simulink model "MinimumJerkPlanner"  (R2024b)
settings: configuration reference "MCConfiguration" (kept outside this file)
undefined symbols (not defined in the file): acc_max, bVelocityMove, InitTrajectory, p0, pos_max, pos_min, target_pos, target_vel, Trajectory_set_pos_end, Trajectory_set_pos_raw, Trajectory_velocity_stop, Ts, vA, vel_max, velAvg, vK0, vK1, vK2, vK3, vK4, vK5, vK6, vT, vTimer, vV, vX, xA, xK0, xK1, xK2, xK3, xK4, xK5, xStar, xT, xTimer, xV, xX
libraries: simulink x4, shareduavrstlib x2
settings Model: DataDictionary=MotionController.sldd  Creator=rpumpo  LastModifiedBy=rpumpo
settings ConfigSetRef: SourceName=MCConfiguration

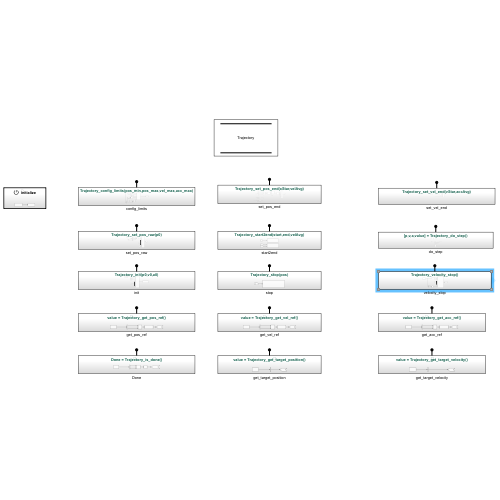
[thumbnail: Simulink's stored preview of the top-level diagram]
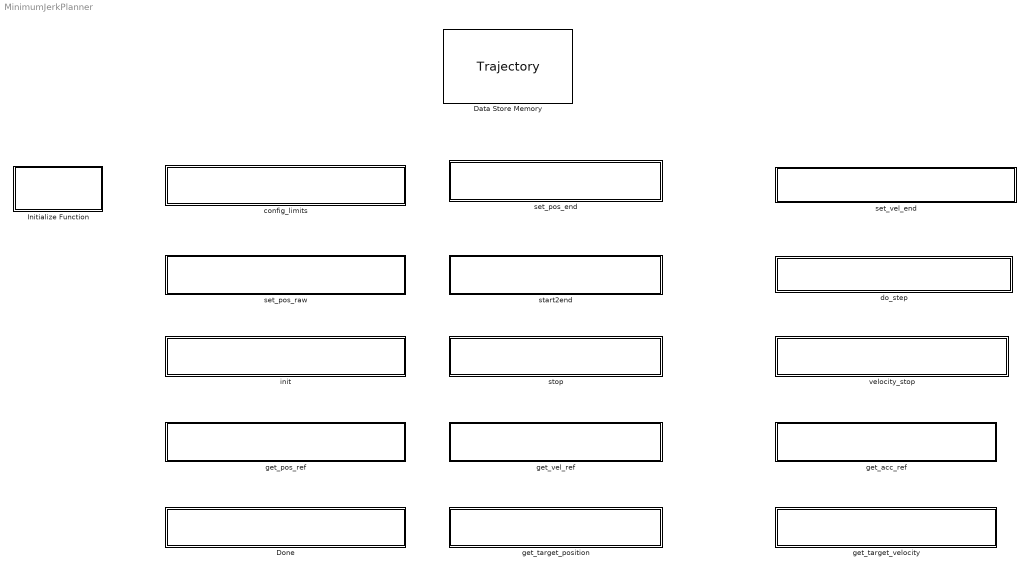
== system MinimumJerkPlanner ==
  Data Store Memory : DataStoreMemory  DataStoreName=Trajectory  WriteAfterWriteMsg=warning  ShowAdditionalParam=off  OutDataTypeStr=Bus: trajectoryhidParameters
  Done : Subsystem  TreatAsAtomicUnit=on
  Initialize Function : Subsystem  TreatAsAtomicUnit=on
  config_limits : Subsystem  TreatAsAtomicUnit=on
  do_step : Subsystem  TreatAsAtomicUnit=on
  get_acc_ref : Subsystem  TreatAsAtomicUnit=on
  get_pos_ref : Subsystem  TreatAsAtomicUnit=on
  get_target_position : Subsystem  TreatAsAtomicUnit=on
  get_target_velocity : Subsystem  TreatAsAtomicUnit=on
  get_vel_ref : Subsystem  TreatAsAtomicUnit=on
  init : Subsystem  TreatAsAtomicUnit=on
  set_pos_end : Subsystem  TreatAsAtomicUnit=on
  set_pos_raw : Subsystem  TreatAsAtomicUnit=on
  set_vel_end : Subsystem  TreatAsAtomicUnit=on
  start2end : Subsystem  TreatAsAtomicUnit=on
  stop : Subsystem  TreatAsAtomicUnit=on
  velocity_stop : Subsystem  TreatAsAtomicUnit=on

== system MinimumJerkPlanner/Done ==
  Trajectory_is_done : TriggerPort  TriggerType=function-call  IsSimulinkFunction=on  FunctionName=Trajectory_is_done  FunctionVisibility=scoped  VariantControl=(inherit)
  Add : Sum  Inputs=+-
  Bus Selector : BusSelector  OutputSignals=xTimer,xT
  Compare To Constant : simulink/Logic and Bit Operations/Compare To Constant  relop=>=  const=0  OutDataTypeStr=boolean
  Data Store Read : DataStoreRead  DataStoreName=Trajectory  IndexOptions=Index vector (dialog)  Indices=1  OutputSizes=1
  Done : ArgOut  OutDataTypeStr=boolean  ArgumentName=Done
  wires:
  Data Store Read/1 -> Bus Selector/1
  Bus Selector/2 -> Add/2  "<xT>"
  Bus Selector/1 -> Add/1  "<xTimer>"
  Add/1 -> Compare To Constant/1
  Compare To Constant/1 -> Done/1

== system MinimumJerkPlanner/Initialize Function ==
  Constant : Constant  Value=InitTrajectory  OutDataTypeStr=Bus: trajectoryhidParameters
  Data Store Write : DataStoreWrite  DataStoreName=Trajectory  IndexOptions=Index vector (dialog)  Indices=1  OutputSizes=1
  Event Listener : EventListener  DisableCoverage=on  EventName=reset
  wires:
  Constant/1 -> Data Store Write/1

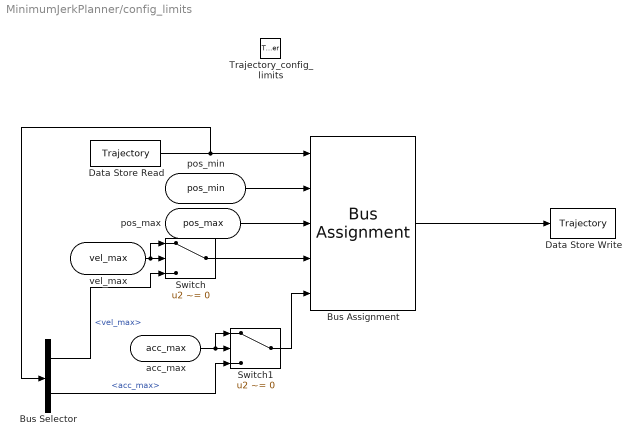
== system MinimumJerkPlanner/config_limits ==
  Trajectory_config_limits : TriggerPort  TriggerType=function-call  IsSimulinkFunction=on  FunctionName=Trajectory_config_limits  FunctionVisibility=scoped  VariantControl=(inherit)
  Bus Assignment : BusAssignment  AssignedSignals=pos_min,pos_max,vel_max,acc_max
  Bus Selector : BusSelector  OutputSignals=vel_max,acc_max
  Data Store Read : DataStoreRead  DataStoreName=Trajectory  IndexOptions=Index vector (dialog)  Indices=1  OutputSizes=1
  Data Store Write : DataStoreWrite  DataStoreName=Trajectory  IndexOptions=Index vector (dialog)  Indices=1  OutputSizes=1
  Switch : Switch  Criteria=u2 ~= 0  SaturateOnIntegerOverflow=off  InputSameDT=off
  Switch1 : Switch  Criteria=u2 ~= 0  SaturateOnIntegerOverflow=off  InputSameDT=off
  pos_min : ArgIn  OutDataTypeStr=single  ArgumentName=pos_min
  pos_max : ArgIn  Port=2  OutDataTypeStr=single  ArgumentName=pos_max
  vel_max : ArgIn  Port=3  OutDataTypeStr=single  ArgumentName=vel_max
  acc_max : ArgIn  Port=4  OutDataTypeStr=single  ArgumentName=acc_max
  wires:
  Data Store Read/1 -> Bus Selector/1, Bus Assignment/1
  pos_min/1 -> Bus Assignment/2
  pos_max/1 -> Bus Assignment/3
  Bus Assignment/1 -> Data Store Write/1
  vel_max/1 -> Switch/1, Switch/2
  Bus Selector/1 -> Switch/3  "<vel_max>"
  Switch/1 -> Bus Assignment/4
  acc_max/1 -> Switch1/1, Switch1/2
  Bus Selector/2 -> Switch1/3  "<acc_max>"
  Switch1/1 -> Bus Assignment/5

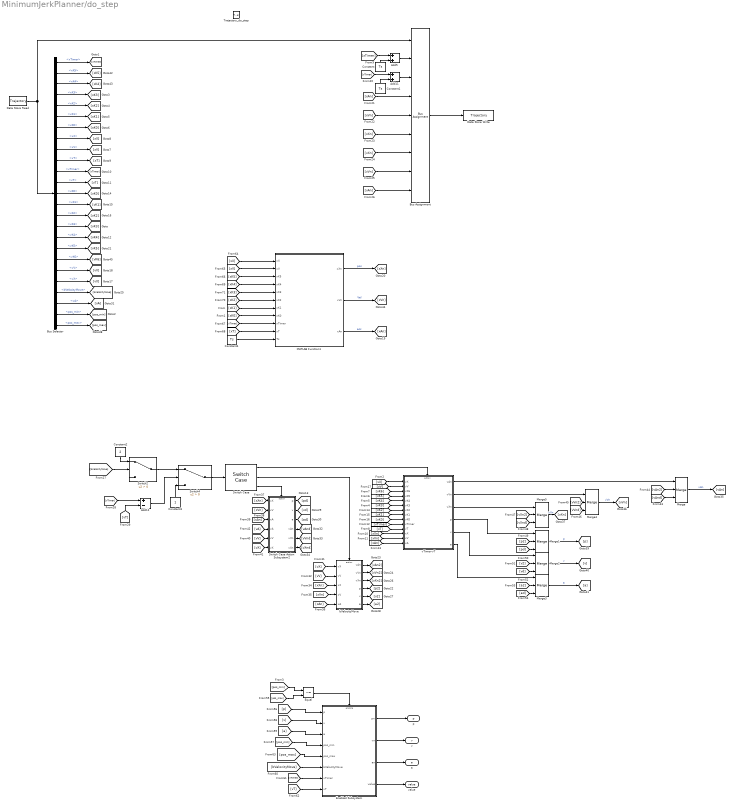
== system MinimumJerkPlanner/do_step ==
  Trajectory_do_step : TriggerPort  TriggerType=function-call  IsSimulinkFunction=on  FunctionName=Trajectory_do_step  FunctionVisibility=scoped  VariantControl=(inherit)
  Add11 : Sum
  Add12 : Sum  Inputs=+-
  Add5 : Sum
  Bus Assignment : BusAssignment  AssignedSignals=xTimer,vTimer,xA,xV,xX,vX,vV,vA
  Bus Selector : BusSelector  OutputSignals=xTimer,xK5,xK4,xK3,xK2,xK1,xK0,xX,xV,xT,vTimer,vT,vK0,vK1,vK2,vK3,vK4,vK5,vK6,vV,vX,bVelocityMove,vA,pos_min,pos_max
  Constant : Constant  Value=Ts  OutDataTypeStr=single
  Constant1 : Constant  Value=Ts  OutDataTypeStr=single
  Constant2 : Constant  Value=2
  Constant3 : Constant
  Constant4 : Constant  Value=Ts  OutDataTypeStr=single
  Data Store Read : DataStoreRead  DataStoreName=Trajectory  IndexOptions=Index vector (dialog)  Indices=1  OutputSizes=1
  Data Store Write : DataStoreWrite  DataStoreName=Trajectory  IndexOptions=Index vector (dialog)  Indices=1  OutputSizes=1
  Enabled Subsystem : Subsystem  TreatAsAtomicUnit=on
  Equal : RelationalOperator  Operator=~=  OutDataTypeStr=boolean  RndMeth=Simplest  InputSameDT=off
  MATLAB Function1 : MATLAB Function  TreatAsAtomicUnit=on
  Merge{,1..5} (6 alike) : Merge  Inputs=3
  Switch Case : SwitchCase  CaseConditions={1,2}
  Switch Case Action Subsystem2 : Subsystem  TreatAsAtomicUnit=on
  Switch2 : Switch  Criteria=u2 > Threshold  SaturateOnIntegerOverflow=off  InputSameDT=off
  Switch4 : Switch  Criteria=u2 > Threshold  SaturateOnIntegerOverflow=off  InputSameDT=off
  bVelocityMove : Subsystem  TreatAsAtomicUnit=on
  vTimer-vT : Subsystem  TreatAsAtomicUnit=on
  p : ArgOut  DisableCoverage=on  OutDataTypeStr=single  ArgumentName=p
  v : ArgOut  DisableCoverage=on  Port=2  OutDataTypeStr=single  ArgumentName=v
  a : ArgOut  DisableCoverage=on  Port=3  OutDataTypeStr=single  ArgumentName=a
  value : ArgOut  DisableCoverage=on  Port=4  OutDataTypeStr=int32  ArgumentName=value
  wires:
  Data Store Read/1 -> Bus Assignment/1, Bus Selector/1
  Bus Selector/1 -> [xTimer]  "<xTimer>"
  Bus Selector/4 -> [xK3]  "<xK3>"
  Bus Selector/5 -> [xK2]  "<xK2>"
  Bus Selector/6 -> [xK1]  "<xK1>"
  Bus Selector/7 -> [xK0]  "<xK0>"
  Bus Selector/8 -> [xX]  "<xX>"
  Bus Selector/9 -> [xV]  "<xV>"
  [xTimer] -> Add5/1
  Constant/1 -> Add5/2
  Add5/1 -> Bus Assignment/2
  Bus Assignment/1 -> Data Store Write/1
  Bus Selector/10 -> [xT]  "<xT>"
  Bus Selector/11 -> [vTimer]  "<vTimer>"
  Bus Selector/12 -> [vT]  "<vT>"
  Bus Selector/13 -> [vK0]  "<vK0>"
  Bus Selector/14 -> [vK1]  "<vK1>"
  Bus Selector/15 -> [vK2]  "<vK2>"
  Bus Selector/20 -> [vV]  "<vV>"
  Bus Selector/21 -> [vX]  "<vX>"
  [xAn] -> Bus Assignment/4
  [xVn] -> Bus Assignment/5
  [xXn] -> Bus Assignment/6
  [vXn] -> Bus Assignment/7
  [vVn] -> Bus Assignment/8
  [vAn] -> Bus Assignment/9
  Bus Selector/22 -> [bVelocityMove]  "<bVelocityMove>"
  [bVelocityMove] -> Switch2/2
  Constant2/1 -> Switch2/1
  Switch Case/1 -> vTimer-vT/Action
  Switch Case/2 -> bVelocityMove/Action
  Switch2/1 -> Switch4/1
  [vX] -> bVelocityMove/1(vX)
  [vV] -> bVelocityMove/2(vV)
  [vTimer] -> Add12/1
  [vT] -> Add12/2
  Add12/1 -> Switch4/2
  Constant3/1 -> Switch4/3
  Switch4/1 -> Switch Case/1
  [vTimer] -> vTimer-vT/10(vTimer)
  [vX] -> vTimer-vT/1(vX)
  [vK2] -> vTimer-vT/7(vK2)
  [vK1] -> vTimer-vT/8(vK1)
  [vK0] -> vTimer-vT/9(vK0)
  [vV] -> vTimer-vT/2(vV)
  [vTimer] -> Add11/1
  Constant1/1 -> Add11/2
  Add11/1 -> Bus Assignment/3
  [xXn] -> bVelocityMove/3(xX)
  [xVn] -> bVelocityMove/4(xV)
  [xAn] -> bVelocityMove/5(xA)
  Switch Case/3 -> Switch Case Action Subsystem2/Action
  [xXn] -> Switch Case Action Subsystem2/1(xX)
  [xVn] -> Switch Case Action Subsystem2/2(xV)
  [xAn] -> Switch Case Action Subsystem2/3(xA)
  Merge/1 -> [vAn]  "vAn"
  Merge1/1 -> [p]  "p"
  [vV] -> Switch Case Action Subsystem2/5(vV)
  [vX] -> Switch Case Action Subsystem2/6(vX)
  [vA] -> Switch Case Action Subsystem2/4(vA)
  Switch Case Action Subsystem2/1(p) -> [pd]
  bVelocityMove/4(p) -> [p2]
  vTimer-vT/4(p) -> Merge1/1
  vTimer-vT/5(v) -> Merge2/1
  vTimer-vT/6(a) -> Merge3/1
  bVelocityMove/6(a) -> [a2]
  bVelocityMove/5(v) -> [v2]
  Switch Case Action Subsystem2/2(v) -> [vd]
  Switch Case Action Subsystem2/3(a) -> [ad]
  Bus Selector/23 -> [vA]  "<vA>"
  vTimer-vT/1(vAn) -> Merge/1
  [vAnd] -> Merge/3
  [vAn2] -> Merge/2
  bVelocityMove/1(vAn) -> [vAn2]
  bVelocityMove/2(vVn) -> [vVn2]
  bVelocityMove/3(vXn) -> [vXn2]
  Switch Case Action Subsystem2/4(vAn) -> [vAnd]
  Switch Case Action Subsystem2/5(vVn) -> [vVnd]
  Switch Case Action Subsystem2/6(vXn) -> [vXnd]
  vTimer-vT/2(vVn) -> Merge4/1
  [vVn2] -> Merge4/2
  [vVnd] -> Merge4/3
  Merge4/1 -> [vVn]  "vVn"
  vTimer-vT/3(vXn) -> Merge5/1
  Merge5/1 -> [vXn]  "vXn"
  [vXn2] -> Merge5/2
  [vXnd] -> Merge5/3
  [p2] -> Merge1/2
  [pd] -> Merge1/3
  [v2] -> Merge2/2
  [vd] -> Merge2/3
  [a2] -> Merge3/2
  [ad] -> Merge3/3
  Bus Selector/24 -> [pos_min]  "<pos_min>"
  Bus Selector/25 -> [pos_max]  "<pos_max>"
  [pos_min] -> Equal/1
  [pos_max] -> Equal/2
  Equal/1 -> Enabled Subsystem/Enable
  [p] -> Enabled Subsystem/1(p)
  [pos_min] -> Enabled Subsystem/4(pos_min)
  Merge2/1 -> [v]  "v"
  Merge3/1 -> [a]  "a"
  [v] -> Enabled Subsystem/2(v)
  [a] -> Enabled Subsystem/3(a)
  [bVelocityMove] -> Enabled Subsystem/6(bVelocityMove)
  [vTimer] -> Enabled Subsystem/7(vTimer)
  [vT] -> Enabled Subsystem/8(vT)
  [pos_max] -> Enabled Subsystem/5(pos_max)
  Enabled Subsystem/2(vn) -> v/1
  Enabled Subsystem/3(an) -> a/1
  Enabled Subsystem/1(pn) -> p/1
  Enabled Subsystem/4(value) -> value/1
  Bus Selector/2 -> [xK5]  "<xK5>"
  Bus Selector/3 -> [xK4]  "<xK4>"
  [xX] -> MATLAB Function1/1(xX)
  [xV] -> MATLAB Function1/2(xV)
  [xK5] -> MATLAB Function1/3(xK5)
  MATLAB Function1/2(xVn) -> [xVn]  "Vel"
  [xTimer] -> MATLAB Function1/9(xTimer)
  [xT] -> MATLAB Function1/10(xT)
  [xK4] -> MATLAB Function1/4(xK4)
  [xK3] -> MATLAB Function1/5(xK3)
  [xK2] -> MATLAB Function1/6(xK2)
  Constant4/1 -> MATLAB Function1/11(Ts)
  [xK1] -> MATLAB Function1/7(xK1)
  [xK0] -> MATLAB Function1/8(xK0)
  MATLAB Function1/3(xAn) -> [xAn]  "acc"
  MATLAB Function1/1(xXn) -> [xXn]  "pos"
  [vK6] -> vTimer-vT/3(vK6)
  [vK5] -> vTimer-vT/4(vK5)
  [vK4] -> vTimer-vT/5(vK4)
  [vK3] -> vTimer-vT/6(vK3)
  [vT] -> vTimer-vT/11(vT)
  [xXn] -> vTimer-vT/12(xX)
  [xVn] -> vTimer-vT/13(xV)
  [xAn] -> vTimer-vT/14(xA)
  Bus Selector/16 -> [vK3]  "<vK3>"
  Bus Selector/17 -> [vK4]  "<vK4>"
  Bus Selector/18 -> [vK5]  "<vK5>"
  Bus Selector/19 -> [vK6]  "<vK6>"

== system MinimumJerkPlanner/get_acc_ref ==
  Trajectory_get_acc_ref : TriggerPort  TriggerType=function-call  IsSimulinkFunction=on  FunctionName=Trajectory_get_acc_ref  FunctionVisibility=scoped  VariantControl=(inherit)
  Add : Sum
  Bus Selector : BusSelector  OutputSignals=xA,vA
  Data Store Read : DataStoreRead  DataStoreName=Trajectory  IndexOptions=Index vector (dialog)  Indices=1  OutputSizes=1
  Data Type Conversion : DataTypeConversion  OutDataTypeStr=int32  SaturateOnIntegerOverflow=off  RndMeth=Floor
  value : ArgOut  OutDataTypeStr=int32  ArgumentName=value
  wires:
  Data Store Read/1 -> Bus Selector/1
  Add/1 -> Data Type Conversion/1
  Data Type Conversion/1 -> value/1
  Bus Selector/1 -> Add/1  "<xA>"
  Bus Selector/2 -> Add/2  "<vA>"

== system MinimumJerkPlanner/get_pos_ref ==
  Trajectory_get_pos_ref : TriggerPort  TriggerType=function-call  IsSimulinkFunction=on  FunctionName=Trajectory_get_pos_ref  FunctionVisibility=scoped  VariantControl=(inherit)
  Add : Sum
  Bus Selector : BusSelector  OutputSignals=xX,vX
  Data Store Read : DataStoreRead  DataStoreName=Trajectory  IndexOptions=Index vector (dialog)  Indices=1  OutputSizes=1
  Data Type Conversion : DataTypeConversion  OutDataTypeStr=int32  SaturateOnIntegerOverflow=off  RndMeth=Floor
  value : ArgOut  OutDataTypeStr=int32  ArgumentName=value
  wires:
  Data Store Read/1 -> Bus Selector/1
  Bus Selector/1 -> Add/1  "<xX>"
  Bus Selector/2 -> Add/2  "<vX>"
  Add/1 -> Data Type Conversion/1
  Data Type Conversion/1 -> value/1

== system MinimumJerkPlanner/get_target_position ==
  Trajectory_get_target_position : TriggerPort  TriggerType=function-call  IsSimulinkFunction=on  FunctionName=Trajectory_get_target_position  FunctionVisibility=scoped  VariantControl=(inherit)
  Bus Selector : BusSelector  OutputSignals=target_pos
  Data Store Read : DataStoreRead  DataStoreName=Trajectory  IndexOptions=Index vector (dialog)  Indices=1  OutputSizes=1
  value : ArgOut  OutDataTypeStr=single  ArgumentName=value
  wires:
  Data Store Read/1 -> Bus Selector/1
  Bus Selector/1 -> value/1  "<target_pos>"

== system MinimumJerkPlanner/get_target_velocity ==
  Trajectory_get_target_velocity : TriggerPort  TriggerType=function-call  IsSimulinkFunction=on  FunctionName=Trajectory_get_target_velocity  FunctionVisibility=scoped  VariantControl=(inherit)
  Bus Selector : BusSelector  OutputSignals=target_vel
  Data Store Read : DataStoreRead  DataStoreName=Trajectory  IndexOptions=Index vector (dialog)  Indices=1  OutputSizes=1
  value : ArgOut  OutDataTypeStr=single  ArgumentName=value
  wires:
  Data Store Read/1 -> Bus Selector/1
  Bus Selector/1 -> value/1  "<target_vel>"

== system MinimumJerkPlanner/get_vel_ref ==
  Trajectory_get_vel_ref : TriggerPort  TriggerType=function-call  IsSimulinkFunction=on  FunctionName=Trajectory_get_vel_ref  FunctionVisibility=scoped  VariantControl=(inherit)
  Add : Sum
  Bus Selector : BusSelector  OutputSignals=xV,vV
  Data Store Read : DataStoreRead  DataStoreName=Trajectory  IndexOptions=Index vector (dialog)  Indices=1  OutputSizes=1
  Data Type Conversion : DataTypeConversion  OutDataTypeStr=int32  SaturateOnIntegerOverflow=off  RndMeth=Floor
  value : ArgOut  OutDataTypeStr=int32  ArgumentName=value
  wires:
  Data Store Read/1 -> Bus Selector/1
  Add/1 -> Data Type Conversion/1
  Data Type Conversion/1 -> value/1
  Bus Selector/1 -> Add/1  "<xV>"
  Bus Selector/2 -> Add/2  "<vV>"

== system MinimumJerkPlanner/init ==
  Trajectory_init : TriggerPort  TriggerType=function-call  IsSimulinkFunction=on  FunctionName=Trajectory_init  FunctionVisibility=scoped  VariantControl=(inherit)
  Bus Assignment : BusAssignment  AssignedSignals=xX,xV,xA,xTimer,xT,vX,vV,vA,vTimer,vT
  Constant : Constant  Value=0  OutDataTypeStr=single
  Data Store Read : DataStoreRead  DataStoreName=Trajectory  IndexOptions=Index vector (dialog)  Indices=1  OutputSizes=1
  Data Store Write : DataStoreWrite  DataStoreName=Trajectory  IndexOptions=Index vector (dialog)  Indices=1  OutputSizes=1
  p0 : ArgIn  OutDataTypeStr=single  ArgumentName=p0
  v0 : ArgIn  Port=2  OutDataTypeStr=single  ArgumentName=v0
  a0 : ArgIn  Port=3  OutDataTypeStr=single  ArgumentName=a0
  wires:
  Data Store Read/1 -> Bus Assignment/1
  p0/1 -> Bus Assignment/2
  v0/1 -> Bus Assignment/3
  a0/1 -> Bus Assignment/4
  Constant/1 -> Bus Assignment/10, Bus Assignment/11, Bus Assignment/9, Bus Assignment/5, Bus Assignment/6, Bus Assignment/7, Bus Assignment/8
  Bus Assignment/1 -> Data Store Write/1

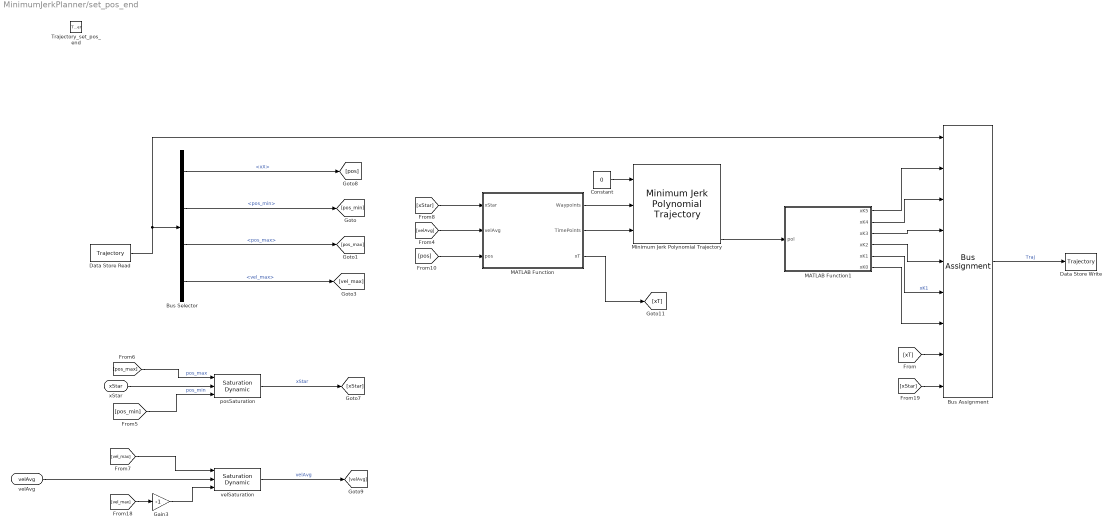
== system MinimumJerkPlanner/set_pos_end ==
  Trajectory_set_pos_end : TriggerPort  TriggerType=function-call  IsSimulinkFunction=on  FunctionName=Trajectory_set_pos_end  FunctionVisibility=scoped  VariantControl=(inherit)
  Bus Assignment : BusAssignment  AssignedSignals=xK5,xK4,xK3,xK2,xK1,xK0,xT,target_pos
  Bus Selector : BusSelector  OutputSignals=xX,pos_min,pos_max,vel_max
  Constant : Constant  Value=0  OutDataTypeStr=single
  Data Store Read : DataStoreRead  DataStoreName=Trajectory  IndexOptions=Index vector (dialog)  Indices=1  OutputSizes=1
  Data Store Write : DataStoreWrite  DataStoreName=Trajectory  IndexOptions=Index vector (dialog)  Indices=1  OutputSizes=1
  Gain3 : Gain  Gain=-1
  MATLAB Function : MATLAB Function  TreatAsAtomicUnit=on
  MATLAB Function1 : MATLAB Function  TreatAsAtomicUnit=on
  Minimum Jerk Polynomial Trajectory : shareduavrstlib/Minimum Jerk Polynomial Trajectory  ShowBCInputPort=off  ShowPolynomialCoefs=on  ShowStatusOutputPort=off  TimeAllocation=off  TimeWeight=100  MinSegmentTime=0.1  MaxSegmentTime=1  MaxIteration=1500  MaxTime=10  SimulateUsing=Code generation
      settings: LibrarySourceBlock=robotutilslib/Minimum Jerk Polynomial Trajectory
  posSaturation : simulink/Discontinuities/Saturation Dynamic  OutMin=[]  OutMax=[]  OutDataTypeStr=Inherit: Same as second input  OutDataType=fixdt(1, 16)  OutScaling=2^-10  DoSatur=off
  velSaturation : simulink/Discontinuities/Saturation Dynamic  OutMin=[]  OutMax=[]  OutDataTypeStr=Inherit: Same as second input  OutDataType=fixdt(1, 16)  OutScaling=2^-10  DoSatur=off
  xStar : ArgIn  DisableCoverage=on  OutDataTypeStr=single  ArgumentName=xStar
  velAvg : ArgIn  DisableCoverage=on  Port=2  OutDataTypeStr=single  ArgumentName=velAvg
  wires:
  [vel_max] -> Gain3/1
  [vel_max] -> velSaturation/1
  Bus Selector/4 -> [vel_max]  "<vel_max>"
  Gain3/1 -> velSaturation/3
  MATLAB Function1/5(xK1) -> Bus Assignment/6  "xK1"
  [pos_min] -> posSaturation/3  "pos_min"
  xStar/1 -> posSaturation/2
  [pos_max] -> posSaturation/1  "pos_max"
  Bus Selector/2 -> [pos_min]  "<pos_min>"
  [xT] -> Bus Assignment/8
  Data Store Read/1 -> Bus Assignment/1, Bus Selector/1
  [xStar] -> Bus Assignment/9
  Bus Assignment/1 -> Data Store Write/1  "Traj"
  posSaturation/1 -> [xStar]  "xStar"
  Bus Selector/1 -> [pos]  "<xX>"
  Bus Selector/3 -> [pos_max]  "<pos_max>"
  velSaturation/1 -> [velAvg]  "velAvg"
  MATLAB Function1/6(xK0) -> Bus Assignment/7
  velAvg/1 -> velSaturation/2
  [velAvg] -> MATLAB Function/2(velAvg)
  [xStar] -> MATLAB Function/1(xStar)
  [pos] -> MATLAB Function/3(pos)
  Constant/1 -> Minimum Jerk Polynomial Trajectory/1
  MATLAB Function/1(Waypoints) -> Minimum Jerk Polynomial Trajectory/2
  MATLAB Function/2(TimePoints) -> Minimum Jerk Polynomial Trajectory/3
  MATLAB Function/3(xT) -> [xT]
  Minimum Jerk Polynomial Trajectory/6 -> MATLAB Function1/1(pol)
  MATLAB Function1/1(xK5) -> Bus Assignment/2
  MATLAB Function1/2(xK4) -> Bus Assignment/3
  MATLAB Function1/3(xK3) -> Bus Assignment/4
  MATLAB Function1/4(xK2) -> Bus Assignment/5

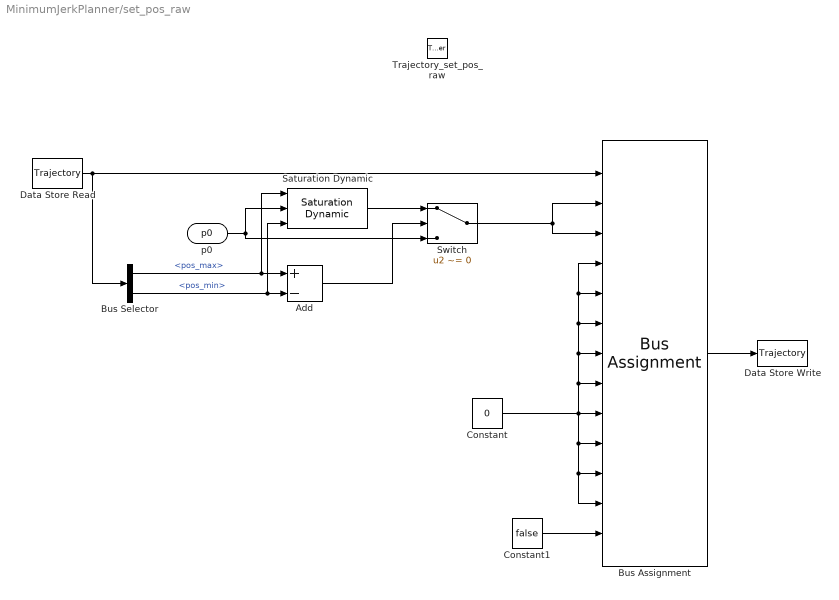
== system MinimumJerkPlanner/set_pos_raw ==
  Trajectory_set_pos_raw : TriggerPort  TriggerType=function-call  IsSimulinkFunction=on  FunctionName=Trajectory_set_pos_raw  FunctionVisibility=scoped  VariantControl=(inherit)
  Add : Sum  Inputs=+-
  Bus Assignment : BusAssignment  AssignedSignals=target_pos,xX,xV,xA,xTimer,xT,vX,vV,vA,vTimer,vT,bVelocityMove
  Bus Selector : BusSelector  OutputSignals=pos_max,pos_min
  Constant : Constant  Value=0  OutDataTypeStr=single
  Constant1 : Constant  Value=false  OutDataTypeStr=boolean
  Data Store Read : DataStoreRead  DataStoreName=Trajectory  IndexOptions=Index vector (dialog)  Indices=1  OutputSizes=1
  Data Store Write : DataStoreWrite  DataStoreName=Trajectory  IndexOptions=Index vector (dialog)  Indices=1  OutputSizes=1
  Saturation Dynamic : simulink/Discontinuities/Saturation Dynamic  OutMin=[]  OutMax=[]  OutDataTypeStr=Inherit: Same as second input  OutDataType=fixdt(1, 16)  OutScaling=2^-10  DoSatur=off
  Switch : Switch  Criteria=u2 ~= 0  SaturateOnIntegerOverflow=off  InputSameDT=off
  p0 : ArgIn  OutDataTypeStr=single  ArgumentName=p0
  wires:
  Bus Assignment/1 -> Data Store Write/1
  Data Store Read/1 -> Bus Assignment/1, Bus Selector/1
  Add/1 -> Switch/2
  Saturation Dynamic/1 -> Switch/1
  p0/1 -> Switch/3, Saturation Dynamic/2
  Switch/1 -> Bus Assignment/2, Bus Assignment/3
  Bus Selector/2 -> Saturation Dynamic/3, Add/2  "<pos_min>"
  Bus Selector/1 -> Saturation Dynamic/1, Add/1  "<pos_max>"
  Constant/1 -> Bus Assignment/5, Bus Assignment/4, Bus Assignment/6, Bus Assignment/7, Bus Assignment/8, Bus Assignment/10, Bus Assignment/11, Bus Assignment/12, Bus Assignment/9
  Constant1/1 -> Bus Assignment/13

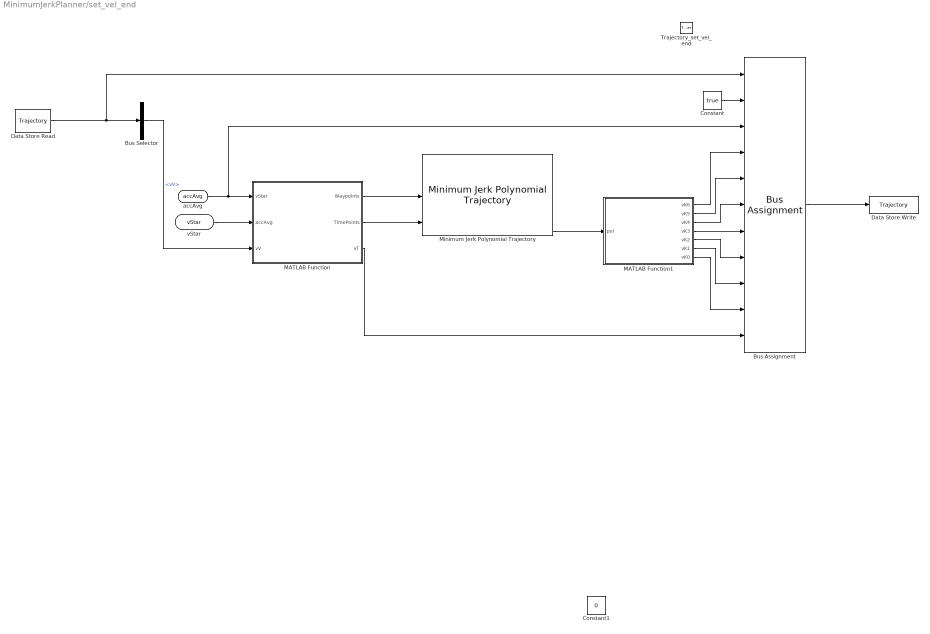
== system MinimumJerkPlanner/set_vel_end ==
  Trajectory_set_vel_end : TriggerPort  TriggerType=function-call  IsSimulinkFunction=on  FunctionName=Trajectory_set_vel_end  FunctionVisibility=scoped  VariantControl=(inherit)
  Bus Assignment : BusAssignment  AssignedSignals=bVelocityMove,target_vel,vK6,vK5,vK4,vK3,vK2,vK1,vK0,vT
  Bus Selector : BusSelector  OutputSignals=vV
  Constant : Constant  Value=true  OutDataTypeStr=boolean
  Constant1 : Constant  Value=0  OutDataTypeStr=single
  Data Store Read : DataStoreRead  DataStoreName=Trajectory  IndexOptions=Index vector (dialog)  Indices=1  OutputSizes=1
  Data Store Write : DataStoreWrite  DataStoreName=Trajectory  IndexOptions=Index vector (dialog)  Indices=1  OutputSizes=1
  MATLAB Function : MATLAB Function  TreatAsAtomicUnit=on
  MATLAB Function1 : MATLAB Function  TreatAsAtomicUnit=on
  Minimum Jerk Polynomial Trajectory : shareduavrstlib/Minimum Jerk Polynomial Trajectory  ShowBCInputPort=off  ShowPolynomialCoefs=on  ShowStatusOutputPort=off  TimeAllocation=off  TimeWeight=100  MinSegmentTime=0.1  MaxSegmentTime=1  MaxIteration=1500  MaxTime=10  SimulateUsing=Code generation
      settings: LibrarySourceBlock=robotutilslib/Minimum Jerk Polynomial Trajectory
  vStar : ArgIn  OutDataTypeStr=single  ArgumentName=vStar
  accAvg : ArgIn  Port=2  OutDataTypeStr=single  ArgumentName=accAvg
  wires:
  Data Store Read/1 -> Bus Assignment/1, Bus Selector/1
  Bus Assignment/1 -> Data Store Write/1
  Constant/1 -> Bus Assignment/2
  accAvg/1 -> Bus Assignment/3, MATLAB Function/1(vStar)
  vStar/1 -> MATLAB Function/2(accAvg)
  Minimum Jerk Polynomial Trajectory/6 -> MATLAB Function1/1(pol)
  MATLAB Function/3(vT) -> Bus Assignment/11
  Bus Selector/1 -> MATLAB Function/3(vV)  "<vV>"
  MATLAB Function/1(Waypoints) -> Minimum Jerk Polynomial Trajectory/2
  MATLAB Function/2(TimePoints) -> Minimum Jerk Polynomial Trajectory/3
  MATLAB Function1/7(vK0) -> Bus Assignment/10
  MATLAB Function1/6(vK1) -> Bus Assignment/9
  MATLAB Function1/5(vK2) -> Bus Assignment/8
  MATLAB Function1/4(vK3) -> Bus Assignment/7
  MATLAB Function1/3(vK4) -> Bus Assignment/6
  MATLAB Function1/2(vK5) -> Bus Assignment/5
  MATLAB Function1/1(vK6) -> Bus Assignment/4

== system MinimumJerkPlanner/start2end ==
  Trajectory_start2end : TriggerPort  TriggerType=function-call  IsSimulinkFunction=on  FunctionName=Trajectory_start2end  FunctionVisibility=scoped  VariantControl=(inherit)
  Function Caller : FunctionCaller  FunctionPrototype=Trajectory_set_pos_raw(p0)  InputArgumentSpecifications=<Enter example>  OutputArgumentSpecifications=<Enter example>
  Function Caller2 : FunctionCaller  FunctionPrototype=Trajectory_set_pos_end(xStar,velAvg)  InputArgumentSpecifications=<Enter example>  OutputArgumentSpecifications=<Enter example>
  start : ArgIn  OutDataTypeStr=single  ArgumentName=start
  end : ArgIn  Port=2  OutDataTypeStr=single  ArgumentName=end
  velAvg : ArgIn  Port=3  OutDataTypeStr=single  ArgumentName=velAvg
  wires:
  start/1 -> Function Caller/1
  end/1 -> Function Caller2/1
  velAvg/1 -> Function Caller2/2

== system MinimumJerkPlanner/stop ==
  Trajectory_stop : TriggerPort  TriggerType=function-call  IsSimulinkFunction=on  FunctionName=Trajectory_stop  FunctionVisibility=scoped  VariantControl=(inherit)
  Function Caller4 : FunctionCaller  FunctionPrototype=Trajectory_set_pos_raw(p0)  InputArgumentSpecifications=<Enter example>  OutputArgumentSpecifications=<Enter example>
  pos : ArgIn  OutDataTypeStr=single  ArgumentName=pos
  wires:
  pos/1 -> Function Caller4/1

== system MinimumJerkPlanner/velocity_stop ==
  Trajectory_velocity_stop : TriggerPort  TriggerType=function-call  IsSimulinkFunction=on  FunctionName=Trajectory_velocity_stop  FunctionVisibility=scoped  VariantControl=(inherit)
  Add : Sum
  Bus Assignment : BusAssignment  AssignedSignals=bVelocityMove,vTimer,vT,vX,vV,vA,target_vel,xX
  Bus Selector : BusSelector  OutputSignals=xX,vX
  Data Store Read : DataStoreRead  DataStoreName=Trajectory  IndexOptions=Index vector (dialog)  Indices=1  OutputSizes=1
  Data Store Write : DataStoreWrite  DataStoreName=Trajectory  IndexOptions=Index vector (dialog)  Indices=1  OutputSizes=1
  Zero : Constant  Value=false  OutDataTypeStr=boolean
  Zero1 : Constant  Value=0  OutDataTypeStr=single
  wires:
  Bus Assignment/1 -> Data Store Write/1
  Data Store Read/1 -> Bus Assignment/1, Bus Selector/1
  Zero/1 -> Bus Assignment/2
  Zero1/1 -> Bus Assignment/8, Bus Assignment/7, Bus Assignment/6, Bus Assignment/4, Bus Assignment/3, Bus Assignment/5
  Bus Selector/2 -> Add/2  "<vX>"
  Bus Selector/1 -> Add/1  "<xX>"
  Add/1 -> Bus Assignment/9

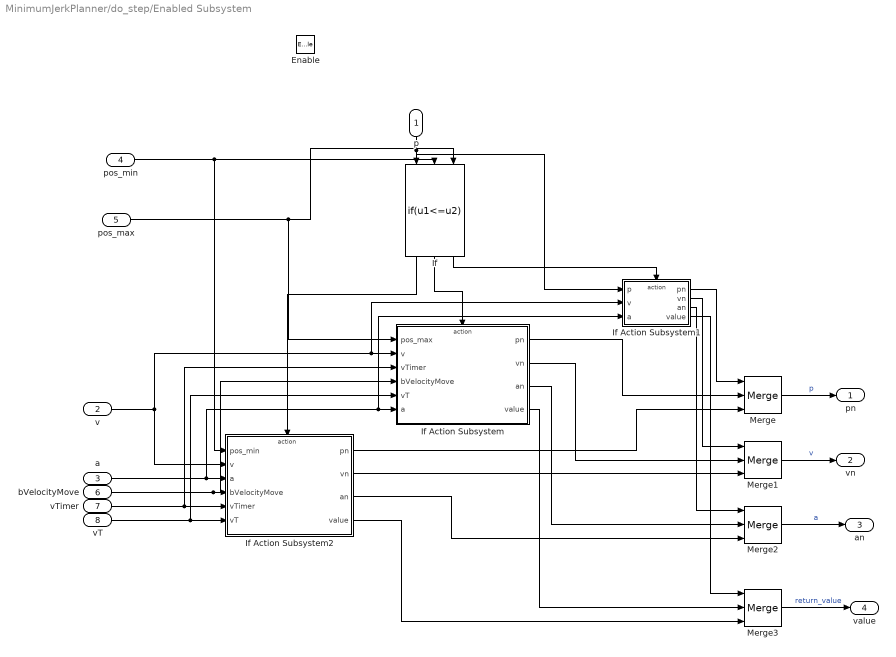
== system MinimumJerkPlanner/do_step/Enabled Subsystem ==
  p : Inport
  v : Inport  Port=2
  a : Inport  Port=3
  pos_min : Inport  Port=4
  pos_max : Inport  Port=5
  bVelocityMove : Inport  Port=6
  vTimer : Inport  Port=7
  vT : Inport  Port=8
  Enable : EnablePort
  If : If  NumInputs=3  IfExpression=u1<=u2  ElseIfExpressions=u1>=u3
  If Action Subsystem : Subsystem  TreatAsAtomicUnit=on
  If Action Subsystem1 : Subsystem  TreatAsAtomicUnit=on
  If Action Subsystem2 : Subsystem  TreatAsAtomicUnit=on
  Merge{,1..3} (4 alike) : Merge  Inputs=3
  pn : Outport
  vn : Outport  Port=2
  an : Outport  Port=3
  value : Outport  Port=4  OutDataTypeStr=int32
  wires:
  pos_min/1 -> If Action Subsystem2/1(pos_min), If/2
  p/1 -> If Action Subsystem1/1(p), If/1
  v/1 -> If Action Subsystem1/2(v), If Action Subsystem/2(v), If Action Subsystem2/2(v)
  bVelocityMove/1 -> If Action Subsystem/4(bVelocityMove), If Action Subsystem2/4(bVelocityMove)
  vTimer/1 -> If Action Subsystem2/5(vTimer), If Action Subsystem/3(vTimer)
  vT/1 -> If Action Subsystem/5(vT), If Action Subsystem2/6(vT)
  a/1 -> If Action Subsystem1/3(a), If Action Subsystem/6(a), If Action Subsystem2/3(a)
  If/1 -> If Action Subsystem2/Action
  If/2 -> If Action Subsystem/Action
  pos_max/1 -> If Action Subsystem/1(pos_max), If/3
  If/3 -> If Action Subsystem1/Action
  If Action Subsystem1/1(pn) -> Merge/1
  If Action Subsystem/1(pn) -> Merge/2
  If Action Subsystem2/1(pn) -> Merge/3
  Merge/1 -> pn/1  "p"
  Merge1/1 -> vn/1  "v"
  If Action Subsystem1/2(vn) -> Merge1/1
  If Action Subsystem/2(vn) -> Merge1/2
  If Action Subsystem2/2(vn) -> Merge1/3
  If Action Subsystem1/3(an) -> Merge2/1
  If Action Subsystem/3(an) -> Merge2/2
  If Action Subsystem2/3(an) -> Merge2/3
  Merge2/1 -> an/1  "a"
  Merge3/1 -> value/1  "return_value"
  If Action Subsystem1/4(value) -> Merge3/1
  If Action Subsystem/4(value) -> Merge3/2
  If Action Subsystem2/4(value) -> Merge3/3

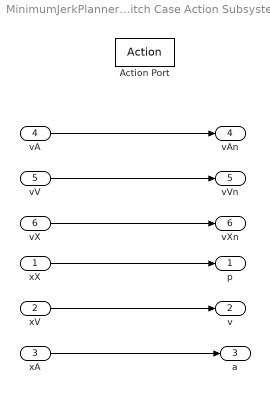
== system MinimumJerkPlanner/do_step/Switch Case Action Subsystem2 ==
  xX : Inport
  xV : Inport  Port=2
  xA : Inport  Port=3
  vA : Inport  Port=4
  vV : Inport  Port=5
  vX : Inport  Port=6
  Action Port : ActionPort  ActionPortLabel=default:
  p : Outport
  v : Outport  Port=2
  a : Outport  Port=3
  vAn : Outport  Port=4
  vVn : Outport  Port=5
  vXn : Outport  Port=6
  wires:
  xX/1 -> p/1
  xV/1 -> v/1
  xA/1 -> a/1
  vA/1 -> vAn/1
  vV/1 -> vVn/1
  vX/1 -> vXn/1

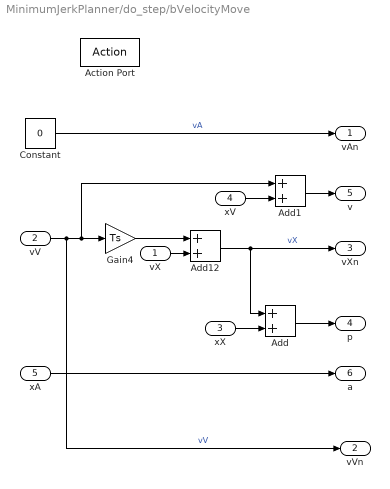
== system MinimumJerkPlanner/do_step/bVelocityMove ==
  vX : Inport
  vV : Inport  Port=2
  xX : Inport  Port=3
  xV : Inport  Port=4
  xA : Inport  Port=5
  Action Port : ActionPort  ActionPortLabel=case [ 2 ]:
  Add : Sum
  Add1 : Sum
  Add12 : Sum
  Constant : Constant  Value=0  OutDataTypeStr=single
  Gain4 : Gain  Gain=Ts
  vAn : Outport
  vVn : Outport  Port=2
  vXn : Outport  Port=3
  p : Outport  Port=4
  v : Outport  Port=5
  a : Outport  Port=6
  wires:
  vX/1 -> Add12/2
  Gain4/1 -> Add12/1
  Add12/1 -> Add/1, vXn/1  "vX"
  vV/1 -> vVn/1, Add1/1, Gain4/1  "vV"
  xA/1 -> a/1
  Constant/1 -> vAn/1  "vA"
  xV/1 -> Add1/2
  Add/1 -> p/1
  xX/1 -> Add/2
  Add1/1 -> v/1

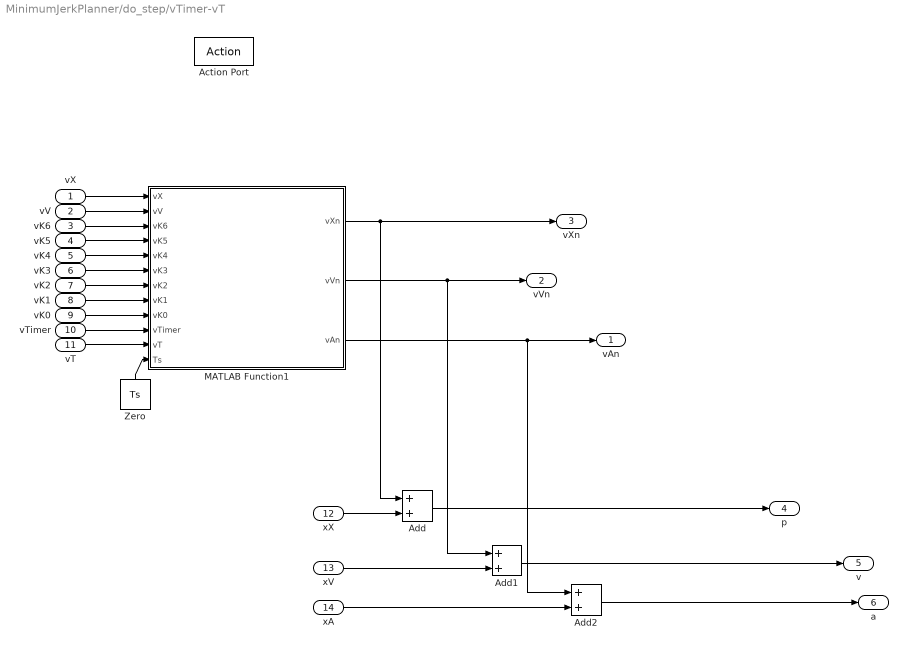
== system MinimumJerkPlanner/do_step/vTimer-vT ==
  vX : Inport
  vV : Inport  Port=2
  vK6 : Inport  Port=3
  vK5 : Inport  Port=4
  vK4 : Inport  Port=5
  vK3 : Inport  Port=6
  vK2 : Inport  Port=7
  vK1 : Inport  Port=8
  vK0 : Inport  Port=9
  vTimer : Inport  Port=10
  vT : Inport  Port=11
  xX : Inport  Port=12
  xV : Inport  Port=13
  xA : Inport  Port=14
  Action Port : ActionPort  ActionPortLabel=case [ 1 ]:
  Add : Sum
  Add1 : Sum
  Add2 : Sum
  MATLAB Function1 : MATLAB Function  TreatAsAtomicUnit=on
  Zero : Constant  Value=Ts  OutDataTypeStr=single
  vAn : Outport
  vVn : Outport  Port=2
  vXn : Outport  Port=3
  p : Outport  Port=4
  v : Outport  Port=5
  a : Outport  Port=6
  wires:
  Zero/1 -> MATLAB Function1/12(Ts)
  vT/1 -> MATLAB Function1/11(vT)
  vTimer/1 -> MATLAB Function1/10(vTimer)
  vK0/1 -> MATLAB Function1/9(vK0)
  vK1/1 -> MATLAB Function1/8(vK1)
  vK2/1 -> MATLAB Function1/7(vK2)
  vK3/1 -> MATLAB Function1/6(vK3)
  vK4/1 -> MATLAB Function1/5(vK4)
  vK5/1 -> MATLAB Function1/4(vK5)
  vK6/1 -> MATLAB Function1/3(vK6)
  vV/1 -> MATLAB Function1/2(vV)
  vX/1 -> MATLAB Function1/1(vX)
  MATLAB Function1/1(vXn) -> vXn/1, Add/1
  MATLAB Function1/2(vVn) -> Add1/1, vVn/1
  MATLAB Function1/3(vAn) -> Add2/1, vAn/1
  xX/1 -> Add/2
  xV/1 -> Add1/2
  xA/1 -> Add2/2
  Add/1 -> p/1
  Add1/1 -> v/1
  Add2/1 -> a/1

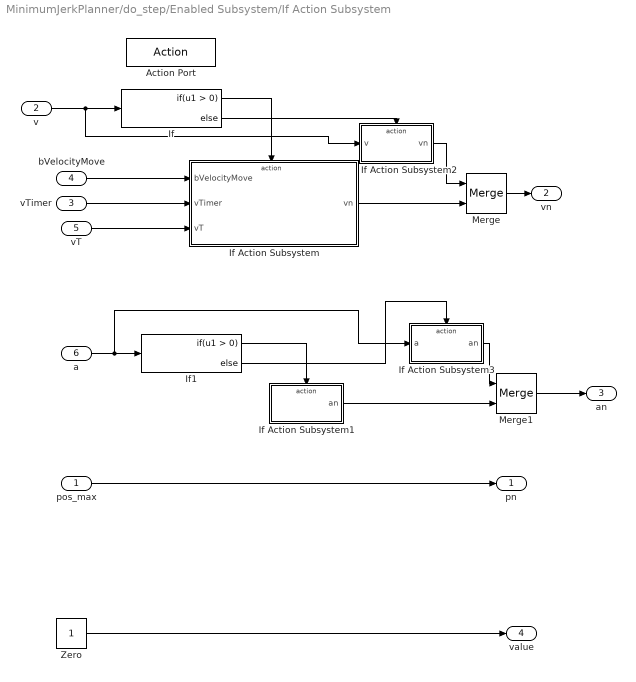
== system MinimumJerkPlanner/do_step/Enabled Subsystem/If Action Subsystem ==
  pos_max : Inport
  v : Inport  Port=2
  vTimer : Inport  Port=3
  bVelocityMove : Inport  Port=4
  vT : Inport  Port=5
  a : Inport  Port=6
  Action Port : ActionPort  ActionPortLabel=elseif(u1>=u3)
  If : If
  If Action Subsystem : Subsystem  TreatAsAtomicUnit=on
  If Action Subsystem1 : Subsystem  TreatAsAtomicUnit=on
  If Action Subsystem2 : Subsystem  TreatAsAtomicUnit=on
  If Action Subsystem3 : Subsystem  TreatAsAtomicUnit=on
  If1 : If
  Merge : Merge
  Merge1 : Merge
  Zero : Constant  OutDataTypeStr=int32
  pn : Outport
  vn : Outport  Port=2
  an : Outport  Port=3
  value : Outport  Port=4
  wires:
  v/1 -> If Action Subsystem2/1(v), If/1
  bVelocityMove/1 -> If Action Subsystem/1(bVelocityMove)
  vTimer/1 -> If Action Subsystem/2(vTimer)
  vT/1 -> If Action Subsystem/3(vT)
  If1/1 -> If Action Subsystem1/Action
  a/1 -> If Action Subsystem3/1(a), If1/1
  pos_max/1 -> pn/1
  Zero/1 -> value/1
  If/1 -> If Action Subsystem/Action
  If/2 -> If Action Subsystem2/Action
  If Action Subsystem2/1(vn) -> Merge/1
  If Action Subsystem/1(vn) -> Merge/2
  Merge/1 -> vn/1
  If1/2 -> If Action Subsystem3/Action
  Merge1/1 -> an/1
  If Action Subsystem3/1(an) -> Merge1/1
  If Action Subsystem1/1(an) -> Merge1/2

== system MinimumJerkPlanner/do_step/Enabled Subsystem/If Action Subsystem1 ==
  p : Inport
  v : Inport  Port=2
  a : Inport  Port=3
  Action Port : ActionPort  ActionPortLabel=else
  Zero : Constant  Value=0  OutDataTypeStr=int32
  pn : Outport
  vn : Outport  Port=2
  an : Outport  Port=3
  value : Outport  Port=4
  wires:
  Zero/1 -> value/1
  p/1 -> pn/1
  a/1 -> an/1
  v/1 -> vn/1

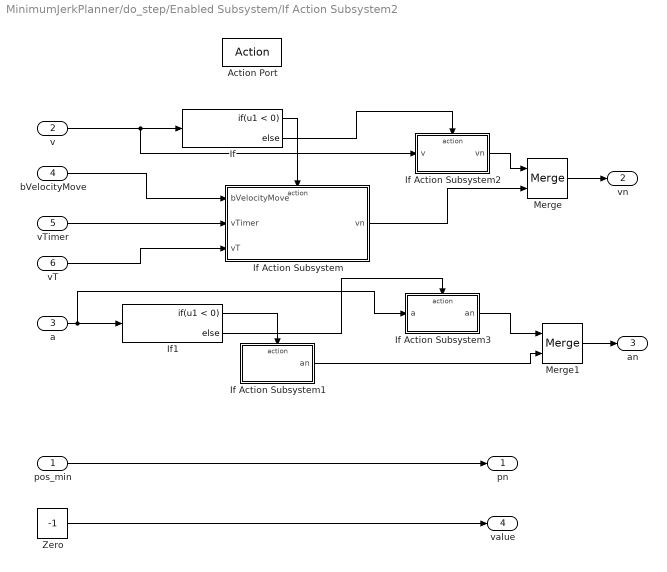
== system MinimumJerkPlanner/do_step/Enabled Subsystem/If Action Subsystem2 ==
  pos_min : Inport
  v : Inport  Port=2
  a : Inport  Port=3
  bVelocityMove : Inport  Port=4
  vTimer : Inport  Port=5
  vT : Inport  Port=6
  Action Port : ActionPort  ActionPortLabel=if(u1<=u2)
  If : If  IfExpression=u1 < 0
  If Action Subsystem : Subsystem  TreatAsAtomicUnit=on
  If Action Subsystem1 : Subsystem  TreatAsAtomicUnit=on
  If Action Subsystem2 : Subsystem  TreatAsAtomicUnit=on
  If Action Subsystem3 : Subsystem  TreatAsAtomicUnit=on
  If1 : If  IfExpression=u1 < 0
  Merge : Merge
  Merge1 : Merge
  Zero : Constant  Value=-1  OutDataTypeStr=int32
  pn : Outport
  vn : Outport  Port=2
  an : Outport  Port=3
  value : Outport  Port=4
  wires:
  pos_min/1 -> pn/1
  bVelocityMove/1 -> If Action Subsystem/1(bVelocityMove)
  a/1 -> If Action Subsystem3/1(a), If1/1
  v/1 -> If Action Subsystem2/1(v), If/1
  vT/1 -> If Action Subsystem/3(vT)
  Zero/1 -> value/1
  vTimer/1 -> If Action Subsystem/2(vTimer)
  If Action Subsystem1/1(an) -> Merge1/2
  If Action Subsystem/1(vn) -> Merge/2
  If1/1 -> If Action Subsystem1/Action
  If/1 -> If Action Subsystem/Action
  If/2 -> If Action Subsystem2/Action
  If Action Subsystem2/1(vn) -> Merge/1
  Merge/1 -> vn/1
  If1/2 -> If Action Subsystem3/Action
  If Action Subsystem3/1(an) -> Merge1/1
  Merge1/1 -> an/1

== system MinimumJerkPlanner/do_step/Enabled Subsystem/If Action Subsystem/If Action Subsystem ==
  bVelocityMove : Inport
  vTimer : Inport  Port=2
  vT : Inport  Port=3
  Action Port : ActionPort  ActionPortLabel=if(u1 > 0)
  Constant : Constant  Value=0  OutDataTypeStr=single
  If : If  IfExpression=u1 ~= 0  ShowElse=off
  If Action Subsystem : Subsystem  TreatAsAtomicUnit=on
  Less Than : RelationalOperator  Operator=<  OutDataTypeStr=boolean  RndMeth=Simplest  InputSameDT=off
  OR : Logic  Operator=OR  IconShape=distinctive  AllPortsSameDT=off  OutDataTypeStr=boolean
  vn : Outport
  wires:
  Constant/1 -> vn/1
  bVelocityMove/1 -> OR/1
  vTimer/1 -> Less Than/1
  vT/1 -> Less Than/2
  Less Than/1 -> OR/2
  OR/1 -> If/1
  If/1 -> If Action Subsystem/Action

== system MinimumJerkPlanner/do_step/Enabled Subsystem/If Action Subsystem/If Action Subsystem1 ==
  Action Port : ActionPort  ActionPortLabel=if(u1 > 0)
  Constant : Constant  Value=0  OutDataTypeStr=single
  an : Outport
  wires:
  Constant/1 -> an/1

== system MinimumJerkPlanner/do_step/Enabled Subsystem/If Action Subsystem/If Action Subsystem2 ==
  v : Inport
  Action Port : ActionPort  ActionPortLabel=else
  vn : Outport
  wires:
  v/1 -> vn/1

== system MinimumJerkPlanner/do_step/Enabled Subsystem/If Action Subsystem/If Action Subsystem3 ==
  a : Inport
  Action Port : ActionPort  ActionPortLabel=else
  an : Outport
  wires:
  a/1 -> an/1

== system MinimumJerkPlanner/do_step/Enabled Subsystem/If Action Subsystem2/If Action Subsystem ==
  bVelocityMove : Inport
  vTimer : Inport  Port=2
  vT : Inport  Port=3
  Action Port : ActionPort  ActionPortLabel=if(u1 < 0)
  Constant : Constant  Value=0  OutDataTypeStr=single
  If : If  IfExpression=u1 ~= 0  ShowElse=off
  If Action Subsystem : Subsystem  TreatAsAtomicUnit=on
  Less Than : RelationalOperator  Operator=<  OutDataTypeStr=boolean  RndMeth=Simplest  InputSameDT=off
  OR : Logic  Operator=OR  IconShape=distinctive  AllPortsSameDT=off  OutDataTypeStr=boolean
  vn : Outport
  wires:
  Constant/1 -> vn/1
  bVelocityMove/1 -> OR/1
  vTimer/1 -> Less Than/1
  vT/1 -> Less Than/2
  Less Than/1 -> OR/2
  OR/1 -> If/1
  If/1 -> If Action Subsystem/Action

== system MinimumJerkPlanner/do_step/Enabled Subsystem/If Action Subsystem2/If Action Subsystem1 ==
  Action Port : ActionPort  ActionPortLabel=if(u1 < 0)
  Constant : Constant  Value=0  OutDataTypeStr=single
  an : Outport
  wires:
  Constant/1 -> an/1

== system MinimumJerkPlanner/do_step/Enabled Subsystem/If Action Subsystem2/If Action Subsystem2 ==
  v : Inport
  Action Port : ActionPort  ActionPortLabel=else
  vn : Outport
  wires:
  v/1 -> vn/1

== system MinimumJerkPlanner/do_step/Enabled Subsystem/If Action Subsystem2/If Action Subsystem3 ==
  a : Inport
  Action Port : ActionPort  ActionPortLabel=else
  an : Outport
  wires:
  a/1 -> an/1

== system MinimumJerkPlanner/do_step/Enabled Subsystem/If Action Subsystem/If Action Subsystem/If Action Subsystem ==
  Action Port : ActionPort  ActionPortLabel=if(u1 ~= 0)
  Function Caller : FunctionCaller  FunctionPrototype=Trajectory_velocity_stop()  InputArgumentSpecifications=<Enter example>  OutputArgumentSpecifications=<Enter example>

== system MinimumJerkPlanner/do_step/Enabled Subsystem/If Action Subsystem2/If Action Subsystem/If Action Subsystem ==
  Action Port : ActionPort  ActionPortLabel=if(u1 ~= 0)
  Function Caller : FunctionCaller  FunctionPrototype=Trajectory_velocity_stop()  InputArgumentSpecifications=<Enter example>  OutputArgumentSpecifications=<Enter example>

== matlab function MinimumJerkPlanner/set_pos_end/MATLAB Function1 ==
  data: xK5 output; xK4 output; xK3 output; xK2 output; xK1 output; xK0 output; pol input
function [xK5,xK4,xK3,xK2,xK1,xK0]  = extract_coefficients(pol)
xK5 = pol(1,1);
xK4 = single(pol(1,2));
xK3 = single(pol(1,3));
xK2 = single(pol(1,4));
xK1 = single(pol(1,5));
xK0 = single(pol(1,6));
end

== matlab function MinimumJerkPlanner/set_pos_end/MATLAB Function ==
  data: Waypoints output; xStar input; TimePoints output; velAvg input; pos input; xT output
function [Waypoints,TimePoints,xT]  = define_trajectories_parameters(xStar,velAvg,pos)
    D = xStar-pos;
    xT = abs(D/velAvg);
    TimePoints = [0,xT];
    Waypoints = [pos xStar ; 0 0];

== matlab function MinimumJerkPlanner/do_step/MATLAB Function1 ==
  data: xX input; xV input; xXn output; xVn output; xK5 input; xK4 input; xK3 input; xK2 input; xK1 input; xK0 input; xTimer input; xAn output; xT input; Ts input
function [xXn,xVn,xAn]  = step(xX,xV,xK5,xK4,xK3,xK2,xK1,xK0,xTimer,xT,Ts)
if (xTimer<= xT)
    xAn = single(42*xK5*xTimer^5+30*xK4*xTimer^4 + 20*xK3*xTimer^3+12*xK2*xTimer^2+6*xK1*xTimer+2*xK0);
else
    xAn = single(0);
end
xVn = single(xV+xAn*Ts);
xXn = xX+ xVn*Ts;
end

== matlab function MinimumJerkPlanner/set_vel_end/MATLAB Function ==
  data: Waypoints output; vStar input; TimePoints output; accAvg input; vV input; vT output
function [Waypoints,TimePoints,vT]  = compute(vStar, accAvg, vV)
    D = vStar- vV;
    vT = abs(D/accAvg);
    TimePoints = [0,vT];
    Waypoints = [vV vStar ; 0 0];

== matlab function MinimumJerkPlanner/set_vel_end/MATLAB Function1 ==
  data: vK6 output; vK5 output; vK4 output; vK3 output; vK2 output; vK1 output; pol input; vK0 output
function [vK6,vK5,vK4,vK3,vK2, vK1, vK0]  = extract_coefficients(pol)
vK6 = pol(1,1);
vK5 = pol(1,2);
vK4 = pol(1,3);
vK3 = pol(1,4);
vK2 = pol(1,5);
vK1 = pol(1,6);
vK0 = pol(1,7);
end

== matlab function MinimumJerkPlanner/do_step/vTimer-vT/MATLAB Function1 ==
  data: vX input; vV input; vXn output; vVn output; vK6 input; vK5 input; vAn output; vK4 input; vK3 input; vK2 input; vK1 input; vK0 input; vTimer input; vT input; Ts input
function [vXn,vVn,vAn]  = step(vX,vV,vK6,vK5,vK4,vK3,vK2,vK1,vK0,vTimer,vT,Ts)
if vTimer<=vT
    vAn = 7*vK6*vTimer^6+6*vK5*vTimer^5+5*vK4*vTimer^4+4*vK3*vTimer^3+3*vK2*vTimer^2+2*vK1*vTimer+vK0;
   
else 
    vAn = single(0);
end
vVn = single(vV+vAn*Ts);
vXn = single(vX+ vVn*Ts);

end
